simulink model "sim_wmap"  (R2019b)
settings: Solver=ode4  StartTime=0.0  StopTime=Tfin  FixedStep=0.5  RelTol=1e-3  EnableMultiTasking=on
values from neighbouring files (symbols this model uses):
  ea_dot_ref = [0.001745;0;0.04859]    [main_wmap.m]
  hr = diag(ll/2)*hr    [main_regulation.m]    (also in main_wmap.m)
  IJ = inv(J)    [main_regulation.m]    (also in main_wmap.m)
  J = diag([10 9 12]*1e3)    [main_regulation.m]    (also in main_wmap.m = [399 -2.81 -1.31)
  q0 = [0.6853 0.6953 0.1531 0.1531]'    [main_regulation.m]    (also in main_wmap.m = [0;0;1;0])
  thr = 0.3927    [main_wmap.m]
  w0 = [0.53 0.53 0.053]'    [main_regulation.m]    (also in main_wmap.m = [0.1;-0.9;0.12])
undefined symbols (not defined in the file or in its folder): animation_rot
libraries: vrlib x1
settings Model: Creator=carlonovara  LastModifiedBy=carlonovara
settings DataIOCC: SaveFormat=StructureWithTime  ReturnWorkspaceOutputs=off
settings OptimizationCC: LifeSpan=inf
settings DebuggingCC: SFUnexpectedBacktrackingDiag=warning  SFNoUnconditionalDefaultTransitionDiag=warning  SFExecutionAtInitializationDiag=none  ArithmeticOperatorsInVariantConditions=warning
settings HardwareCC: ProdBitPerSizeT=32  ProdBitPerPtrDiffT=32  ProdWordSize=32  ProdHWDeviceType=Specified
settings SFSimCC: SimUseLocalCustomCode=off  CustomCodeUndefinedFunction=UseInterfaceOnly
settings RTWCC: RTWUseLocalCustomCode=off
settings CodeAppCC: StateflowObjectComments=on
settings GRTTargetCC: TargetLangStandard=C89/C90 (ANSI)  GeneratePreprocessorConditionals=Disable all
settings ConfigComp: CovMetricSettings=dw  CovHtmlReporting=on  CovSaveCumulativeToWorkspaceVar=on  CovSaveSingleToWorkspaceVar=on  CovExternalEMLEnable=off

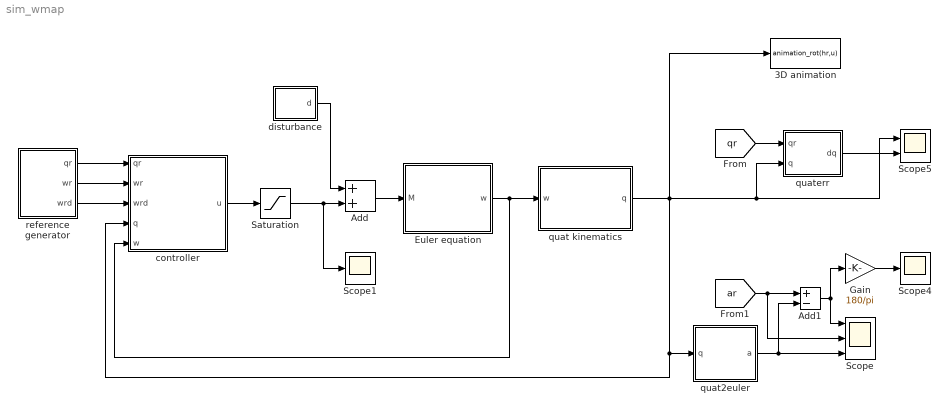
== system sim_wmap ==
  3D animation : MATLABFcn  MATLABFcn=animation_rot(hr,u)  OutputDimensions=0
  Add : Sum
  Add1 : Sum  Inputs=+-
  Euler equation : Subsystem
  Gain : Gain  Gain=180/pi
  Saturation : Saturate  UpperLimit=10  LowerLimit=-10
  Scope : Scope  NumInputPorts=3
  Scope1 : Scope
  Scope4 : Scope
  Scope5 : Scope  NumInputPorts=2
  controller : MATLAB Function  TreatAsAtomicUnit=on
  disturbance : Subsystem
  quat kinematics : Subsystem  AncestorBlock=lib_rotations_2014/quat kinematics
  quat2euler : MATLAB Function  TreatAsAtomicUnit=on
  quaterr : MATLAB Function  TreatAsAtomicUnit=on
  reference generator : Subsystem
  wires:
  Euler equation/1(w) -> quat kinematics/1(w), controller/5(w)
  quat kinematics/1(q) -> controller/4(q), quat2euler/1(q), quaterr/2(q), Scope5/1, 3D animation/1
  reference generator/1(qr) -> controller/1(qr)
  reference generator/2(wr) -> controller/2(wr)
  reference generator/3(wrd) -> controller/3(wrd)
  controller/1(u) -> Saturation/1
  Add/1 -> Euler equation/1(M)
  disturbance/1(d) -> Add/1
  Saturation/1 -> Scope1/1, Add/2
  [qr] -> quaterr/1(qr)
  Add1/1 -> Gain/1, Scope/1
  [ar] -> Add1/1, Scope/2
  quat2euler/1(a) -> Add1/2, Scope/3
  Gain/1 -> Scope4/1
  quaterr/1(dq) -> Scope5/2

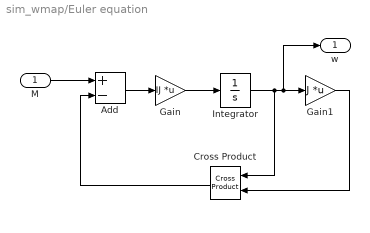
== system sim_wmap/Euler equation ==
  M : Inport
  Add : Sum  Inputs=+-
  Cross Product : vrlib/Utilities/Cross Product
      settings: SourceProductBaseCode=VR
  Gain : Gain  Gain=IJ  Multiplication=Matrix(K*u)
  Gain1 : Gain  Gain=J  Multiplication=Matrix(K*u)
  Integrator : Integrator  InitialCondition=w0
  w : Outport  VectorParamsAs1DForOutWhenUnconnected=off
  wires:
  Cross Product/1 -> Add/2
  Add/1 -> Gain/1
  Gain1/1 -> Cross Product/2
  Gain/1 -> Integrator/1
  Integrator/1 -> Gain1/1, w/1, Cross Product/1
  M/1 -> Add/1

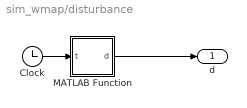
== system sim_wmap/disturbance ==
  Clock : Clock
  MATLAB Function : MATLAB Function  TreatAsAtomicUnit=on
  d : Outport  VectorParamsAs1DForOutWhenUnconnected=off
  wires:
  MATLAB Function/1(d) -> d/1
  Clock/1 -> MATLAB Function/1(t)

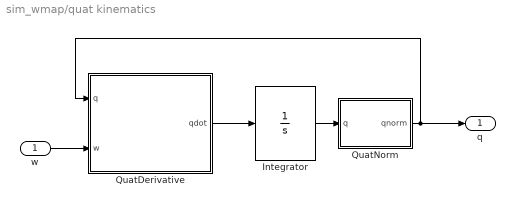
== system sim_wmap/quat kinematics ==
  w : Inport  PortDimensions=3
  Integrator : Integrator  InitialCondition=q0
  QuatDerivative : MATLAB Function  TreatAsAtomicUnit=on
  QuatNorm : MATLAB Function  TreatAsAtomicUnit=on
  q : Outport  PortDimensions=4  VectorParamsAs1DForOutWhenUnconnected=off
  wires:
  w/1 -> QuatDerivative/2(w)
  QuatDerivative/1(qdot) -> Integrator/1
  QuatNorm/1(qnorm) -> QuatDerivative/1(q), q/1
  Integrator/1 -> QuatNorm/1(q)

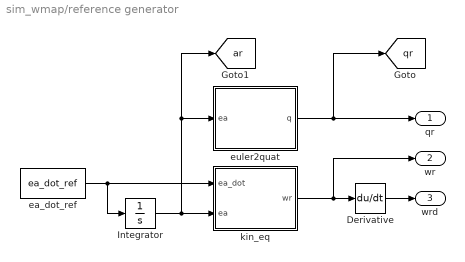
== system sim_wmap/reference generator ==
  Derivative : Derivative
  "Integrator " : Integrator  InitialCondition=[0;thr;0]
  ea_dot_ref : Constant  Value=ea_dot_ref
  "euler2quat " : MATLAB Function  TreatAsAtomicUnit=on
  kin_eq : MATLAB Function  TreatAsAtomicUnit=on
  qr : Outport  VectorParamsAs1DForOutWhenUnconnected=off
  wr : Outport  Port=2  VectorParamsAs1DForOutWhenUnconnected=off
  wrd : Outport  Port=3  VectorParamsAs1DForOutWhenUnconnected=off
  tag scope: ar=global, qr=global
  wires:
  ea_dot_ref/1 -> "Integrator "/1, kin_eq/1(ea_dot)
  kin_eq/1(wr) -> wr/1, Derivative/1
  "euler2quat "/1(q) -> qr/1, [qr]
  Derivative/1 -> wrd/1
  "Integrator "/1 -> [ar], "euler2quat "/1(ea), kin_eq/2(ea)

== matlab function sim_wmap/reference generator/kin_eq ==
  data: ea_dot input; ea input; wr output
function wr = kin_eq(ea_dot,ea)
%#codegen

A=[sin(ea(2))*sin(ea(3)) cos(ea(3)) 0
    sin(ea(2))*cos(ea(3)) -sin(ea(3)) 0
    cos(ea(2)) 0 1];

wr=A*ea_dot;

== matlab function sim_wmap/controller ==
  data: qr input; wr input; wrd input; q input; u output; w input
function u = controller(qr,wr,wrd,q,w)
%#codegen

%J=[399 -2.81 -1.31;-2.81 377 2.54;-1.31 2.54 377];
J=[380 -2.81 -1.31;-2.81 360 2.54;-1.31 2.54 340];

u=zeros(3,1);

qs=[q(1);-q(2:4)];
dq=quatprod(qs,qr);

k1=1;
k2=1;
% u=J*(k2/2*(dq(1)*(wr-w)+0.1*dq(2:4))+wrd)+croprod(w,J*w);
us=J*(k2/2*(dq(1)*(wr-w)+crossprod(dq(2:4),wr+w))+wrd)+crossprod(w,J*w);
% ue=J*(k2/2*(abs(dq(1))*(wr-w)+sign(dq(1))*croprod(dq(2:4),wr+w))+wrd)+croprod(w,J*w);
s=wr-w+k2*dq(2:4);
u=us+k1*J*tanh(1*s);

end

== matlab function sim_wmap/reference generator/euler2quat  ==
  data: ea input; q output
function q = euler2quat(ea)
%#codegen

% case 313
q1=[cos(ea(1)/2);0;0;sin(ea(1)/2)];
q2=[cos(ea(2)/2);sin(ea(2)/2);0;0];
q3=[cos(ea(3)/2);0;0;sin(ea(3)/2)];
q=quatprod(q1,quatprod(q2,q3));

== matlab function sim_wmap/quat2euler ==
  data: q input; a output
function a = quat2euler(q)
%#codegen

T=[q(1)^2+q(2)^2-q(3)^2-q(4)^2 2*(q(2)*q(3)-q(1)*q(4)) 2*(q(2)*q(4)+q(1)*q(3))
    2*(q(2)*q(3)+q(1)*q(4)) q(1)^2-q(2)^2+q(3)^2-q(4)^2 2*(q(3)*q(4)-q(1)*q(2))
    2*(q(2)*q(4)-q(1)*q(3)) 2*(q(3)*q(4)+q(1)*q(2)) q(1)^2-q(2)^2-q(3)^2+q(4)^2];

% 313
a=zeros(3,1);
a(1)=atan2(T(1,3),-T(2,3));
a(2)=atan2(sin(a(1))*T(1,3)-cos(a(1))*T(2,3),T(3,3));
a(3)=atan2(-cos(a(1))*T(1,2)-sin(a(1))*T(2,2),cos(a(1))*T(1,1)+sin(a(1))*T(2,1));

== matlab function sim_wmap/quaterr ==
  data: qr input; dq output; q input
function dq = quterr(qr,q)
%#codegen

qs=[q(1);-q(2:4)];
dq=quatprod(qs,qr);

== matlab function sim_wmap/disturbance/MATLAB Function ==
  data: t input; d output
function d = disturb(t)
%#codegen

d=[0.005*sin(0.05*t)
    0.003
    0.005*cos(0.05*t)];

% d=[0.005*sin(0.1*t)
%     0.005*cos(0.1*t)
%     0.005*cos(0.1*t)];

== matlab function sim_wmap/quat kinematics/QuatDerivative ==
  data: q input; qdot output; w input
function qdot= QuatDerivative(q,w)
%#codegen
omegaq=[0; w];
Q=[q(1) -q(2) -q(3) -q(4);
    q(2) q(1) -q(4) q(3);
    q(3) q(4) q(1) -q(2);
    q(4) -q(3) q(2) q(1)];
qdot=Q*omegaq/2;

== matlab function sim_wmap/quat kinematics/QuatNorm ==
  data: q input; qnorm output
function qnorm = QuatNorm(q)
%#codegen
qnorm=zeros(4,1);
q2=sqrt(q'*q);
qnorm=q/q2;
